simulink model "adrc2"  (Simulink 6.2)
settings: Solver=ode45  StartTime=0.0  StopTime=80.0  RelTol=1e-3
settings Model: LastModifiedBy=lizhijun
settings DebuggingCC: SolverPrmCheckMsg=warning

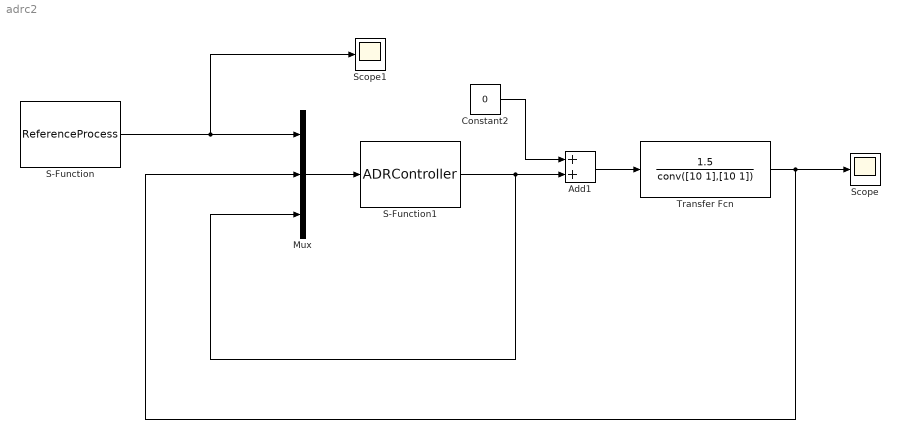
== system adrc2 ==
  Add1 : Sum  OutScaling=2^-10  SampleTime=0.1
  Constant2 : Constant  Value=0
  Mux : Mux  Inputs=3
  S-Function : S-Function  FunctionName=ReferenceProcess  Parameters=SetPoint, RisingTime,SampleTime  mask{SetPoint=1, RisingTime=8, SampleTime=0.1}
  S-Function1 : S-Function  FunctionName=ADRController  Parameters=Beta1,Beta2,Delta1,A1,A2,Delta2,Gamma1,Gamma2,Gamma3,b0,SampleTime  mask{Beta1=100, Beta2=80, Delta1=0.2, A1=3/4, A2=3/2, Delta2=0.5, Gamma1=20, Gamma2=20, Gamma3=30, b0=1.5/100, SampleTime=0.1}
      mask prompts: Beta1 "Proportion Coefficient"; Beta2 "Derivation Coefficient"; Delta1 "Linear Region1 of PID"; A1 "Proportion Power"; A2 "Derivation Power"; Delta2 "Linear Region2 of Observer"; Gamma1 "Observer Coefficient1"; Gamma2 "Observer Coefficient2"; Gamma3 "Observer Coefficient3"; b0 "System Gain"; SampleTime "Sample Time"
  Scope : Scope
      settings: YMin=-4e+014  YMax=5e+014
  Scope1 : Scope
      settings: YMin=2.77556e-017  YMax=1
  Transfer Fcn : TransferFcn  Numerator=[1.5]  Denominator=conv([10 1],[10 1])
  wires:
  S-Function1/1 -> Mux/3, Add1/2
  Transfer Fcn/1 -> Mux/2, Scope/1
  Mux/1 -> S-Function1/1
  S-Function/1 -> Mux/1, Scope1/1
  Constant2/1 -> Add1/1
  Add1/1 -> Transfer Fcn/1
